simulink model "SAME5x_PIM_MCLV2_ioconfig"  (R2020b)
settings: Solver=FixedStepDiscrete  StartTime=0.0  StopTime=10.0  FixedStep=5e-5  RelTol=1e-3  EnableMultiTasking=on
InitFcn:
  | % DC Voltage
  | VDC = 24;
  | 
  | 
  | % QEI
  | lines = 4*1000;
  | p=4;
  | eleclines = lines/p;
  | inveleclines = 1/eleclines
undefined symbols (not defined in the file): AIN0, AIN6, DiscIntNeverNeededParam, gcbh, MCHP_CompilerOptimisation_Callback, MCHP_Master_Callback, MCHP_PDEC_Callback, MCHP_TCC_PWM_Callback, MCHP_UART_Config_Callback, PA02, PA03, PA06, PB08, Pin, VREFA
libraries: simulink x11, MCHP_Blockset x5
(part 3 of 3)

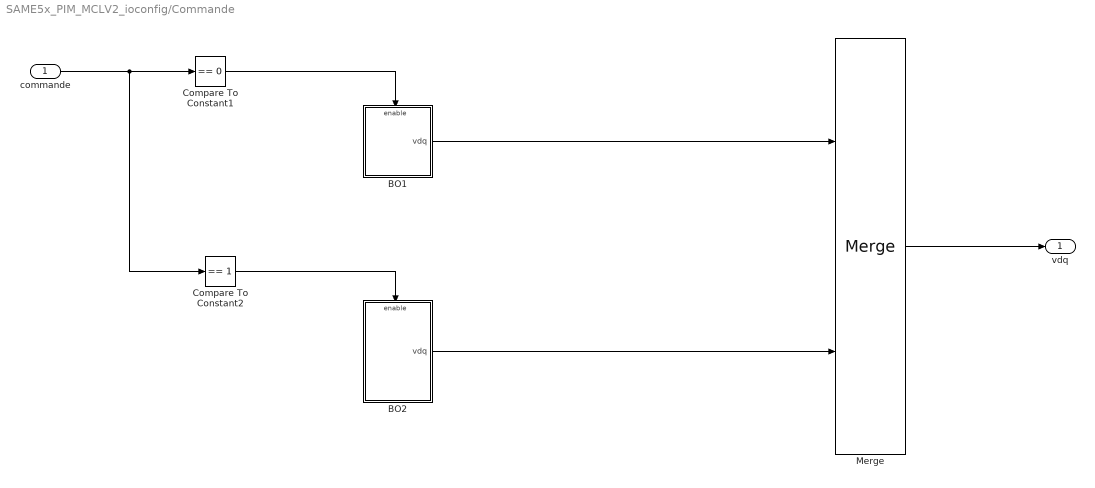
== system SAME5x_PIM_MCLV2_ioconfig/Commande ==
  commande : Inport
  BO1 : Subsystem
  BO2 : Subsystem
  Compare To Constant1 : simulink/Logic and Bit Operations/Compare To Constant  relop===  const=0  OutDataTypeStr=boolean
  Compare To Constant2 : simulink/Logic and Bit Operations/Compare To Constant  relop===  const=1  OutDataTypeStr=boolean
  Merge : Merge
  vdq : Outport  VectorParamsAs1DForOutWhenUnconnected=off
  wires:
  BO2/1(vdq) -> Merge/2
  BO1/1(vdq) -> Merge/1
  Compare To Constant2/1 -> BO2/Enable
  Merge/1 -> vdq/1
  commande/1 -> Compare To Constant2/1, Compare To Constant1/1
  Compare To Constant1/1 -> BO1/Enable

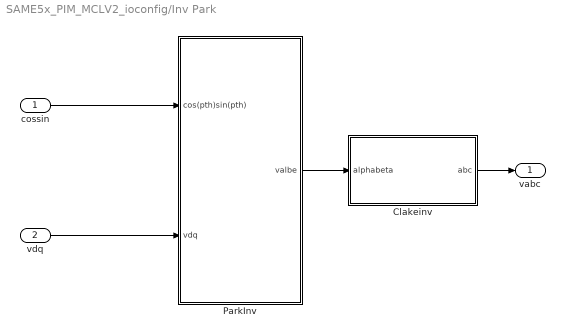
== system SAME5x_PIM_MCLV2_ioconfig/Inv Park ==
  cossin : Inport
  vdq : Inport  Port=2
  Clakeinv : Subsystem
  ParkInv : Subsystem
  vabc : Outport  VectorParamsAs1DForOutWhenUnconnected=off
  wires:
  Clakeinv/1(abc) -> vabc/1
  ParkInv/1(valbe) -> Clakeinv/1(alphabeta)
  cossin/1 -> ParkInv/1(cos(pth)sin(pth))
  vdq/1 -> ParkInv/2(vdq)

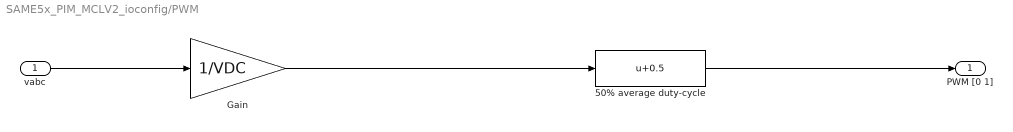
== system SAME5x_PIM_MCLV2_ioconfig/PWM ==
  vabc : Inport
  50% average duty-cycle : Bias  Bias=0.5
  Gain : Gain  Gain=1/VDC  OutDataTypeStr=double
  PWM [0 1] : Outport  VectorParamsAs1DForOutWhenUnconnected=off
  wires:
  Gain/1 -> 50% average duty-cycle/1
  50% average duty-cycle/1 -> PWM [0 1]/1
  vabc/1 -> Gain/1

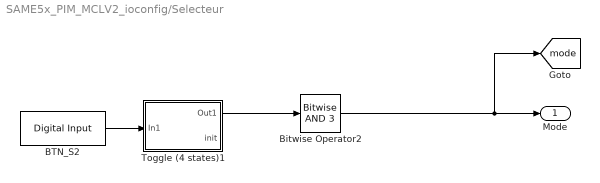
== system SAME5x_PIM_MCLV2_ioconfig/Selecteur ==
  BTN_S2 : MCHP_Blockset/Digital IO/Digital Input  PORT=Dynamic Options  PORT_TXT="D   [ 0  1  8  9  10  11  12  20  21 ]"  PIN=9  PACK=off  SIMULTANEOUS=off  ORDERING=None  SampleTime=.1  MCHP_PORT={Digital In}{DIN}2:0:D9;  MCHP_MASTERLINK=SAME5x_PIM_MCLV2_ioconfig/Microchip Master
      settings: SourceProductName=MPLAB Device Blocks for Simulink
  Bitwise Operator2 : simulink/Logic and Bit Operations/Bitwise Operator  logicop=AND  UseBitMask=on  BitMask=3  BitMaskRealWorld=Stored Integer
  Toggle (4 states)1 : Subsystem
  Mode : Outport  VectorParamsAs1DForOutWhenUnconnected=off
  tag scope: mode=global
  wires:
  BTN_S2/1 -> Toggle (4 states)1/1(In1)
  Toggle (4 states)1/1(Out1) -> Bitwise Operator2/1
  Bitwise Operator2/1 -> [mode], Mode/1

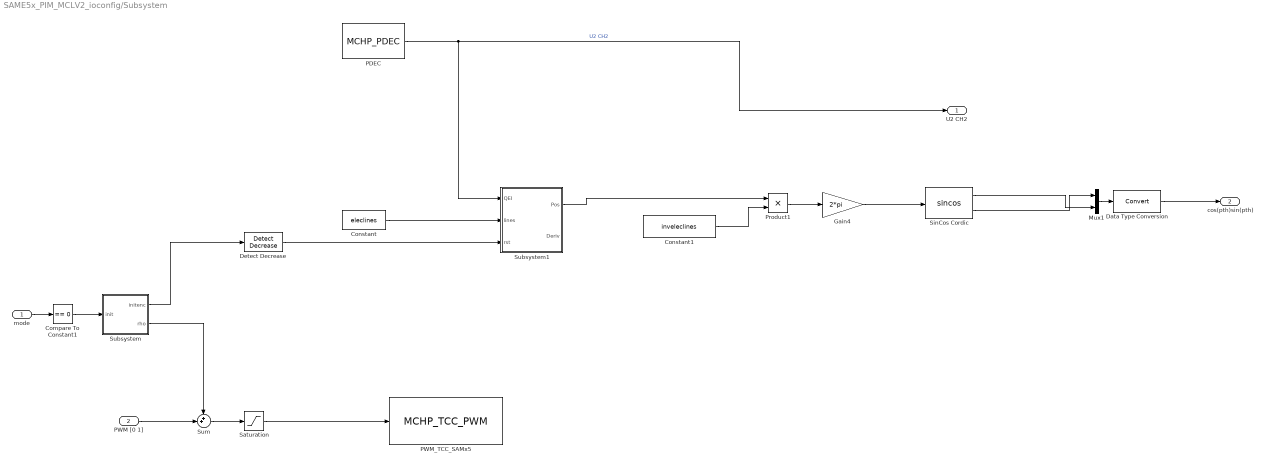
== system SAME5x_PIM_MCLV2_ioconfig/Subsystem ==
  mode : Inport
  PWM [0 1] : Inport  Port=2
  Compare To Constant1 : simulink/Logic and Bit Operations/Compare To Constant  relop===  const=0  OutDataTypeStr=boolean
  Constant : Constant  Value=eleclines
  Constant1 : Constant  Value=inveleclines
  Data Type Conversion : DataTypeConversion
  Detect Decrease : simulink/Logic and Bit Operations/Detect Decrease  vinit=0.0  OutDataTypeStr=boolean
  Gain4 : Gain  Gain=2*pi  OutMin=[0]  OutMax=[2*pi]  OutDataTypeStr=fixdt(0,16)
  Mux1 : Mux  Inputs=2
  PDEC : S-Function  InitFcn=MCHP_PDEC_Callback(gcb,'InitFcn');  FunctionName=MCHP_PDEC  Parameters=MCHP_PDEC_Callback(gcbh,'S_INPUT'),MCHP_PDEC_Callback(gcbh,'S_OUTPUT'),MCHP_PDEC_Callback(gcbh,'S_INPUT_Size'),MCHP_PDEC_Callback(gcbh,'S_OUTPUT_Size'),MCHP_PDEC_Callback(gcbh,'S_ListCustomDatatype'),SampleTime,0  SFunctionDeploymentMode=off  EnableBusSupport=off  mask(PDEC){Mode=Quadrature Encoder, index=Reset counter, QDI0=PC16 / Pin[70] / qdi0, QDI0_txt=Dynamic Options, QDI1=PC17 / Pin[71] / qdi1, QDI1_txt=Dynamic Options, QDI2=PC18 / Pin[72] / qdi2, QDI2_txt=Dynamic Options, maxCounterReset=-1, info=0, MCHP_MASTERLINK=SAME5x_PIM_MCLV2_ioconfig/Microchip Master, SampleTime=1e-4, MCHP_PORT={PDEC A}{PDEC_QDI0}5:0:P80;{PDEC B}{PDEC_QDI1}5:0:P81;{PDEC index}{PDEC_QDI2}5:0:P82;, MAXPOS_INPUT=off, RESET_INPUT=off, OutputCounter=on, OutputRevolution=off, CounterRevolution_length=Counter is 13 bits ; revolution is 3 bits, FILTER=2.55 (us)  ->  freq 196 (KHz), FILTER_TXT=2.55 (us)  ->  freq 196 (KHz), AutoCorrection=on, SWAP=off, QDI_invert_0=off, QDI_invert_1=off, QDI_invert_2=on}
      mask prompts: QDI0 "Phase A (QDI0)"; QDI0_txt "Signal 0"; QDI1 "Phase B (QDO1)"; QDI1_txt "Signal 1"; QDI2 "Index (QDI2)"; QDI2_txt "Signal 2"; maxCounterReset "Reset counter at value (-1 for never)"; SampleTime "Sample Time"; MAXPOS_INPUT "Max Counter is a block input"; RESET_INPUT "Reset Position and Counter on block input level"; OutputCounter "Output counter value"; OutputRevolution "Output revolution"; CounterRevolution_length "Length"; FILTER "Filter: min signal duration"; FILTER_TXT "Filter inputs"; AutoCorrection "Enable Auto-correction"; SWAP "Swap pin phase A && B"; QDI_invert_0 "Invert Phase A logic (QDI0)"; QDI_invert_1 "Invert Phase B logic (QDI1)"; QDI_invert_2 "Invert index logic (QDI2)"
      mask help:
      | PDEC peripheral for SAM D5x / E5x
      |
      | Quadrature Encoder
      mask init:
      | MCHP_PDEC_Callback(gcbh,'INITIALISATION');
      settings: CopyFcn=MCHP_Fun.BlockUpdate(gcbh);  DeleteFcn=MCHP_PDEC_Callback(gcbh,'DeleteFcn')  OpenFcn=MCHP_PDEC_Callback(gcb,'OPEN');
      mask TypeOptions Mode: Quadrature Encoder | Counter with direction
      mask Callback Mode: MCHP_PDEC_Callback(gcbh,'UpdateGUI');
      mask TypeOptions index: Not used | Reset counter
      mask Callback index: MCHP_PDEC_Callback(gcbh,'UpdateGUI');
      mask TypeOptions QDI0: PA24 / Pin[94] / qdi0 | PB18 / Pin[84] / qdi0 | PB23 / Pin[99] / qdi0 | PC16 / Pin[70] / qdi0
      mask TypeOptions QDI0_txt: Dynamic Options
      mask TypeOptions QDI1: PA25 / Pin[95] / qdi1 | PB19 / Pin[85] / qdi1 | PB24 / Pin[100] / qdi1 | PC17 / Pin[71] / qdi1
      mask TypeOptions QDI1_txt: Dynamic Options
      mask TypeOptions QDI2: PB20 / Pin[86] / qdi2 | PB22 / Pin[98] / qdi2 | PB25 / Pin[101] / qdi2 | PC18 / Pin[72] / qdi2
      mask TypeOptions QDI2_txt: Dynamic Options
      mask Callback MAXPOS_INPUT: MCHP_PDEC_Callback(gcbh,'UpdateGUI');
      mask Callback OutputRevolution: MCHP_PDEC_Callback(gcbh,'UpdateGUI');
      mask TypeOptions CounterRevolution_length: Counter is 16 bits ; no revolution | Counter is 15 bits ; revolution is 1 bit | Counter is 14 bits ; revolution is 2 bits | Counter is 13 bits ; revolution is 3 bits | Counter is 12 bits ; revolution is 4 bits | Counter is 11 bits ; revolution is 5 bits | Counter is 10 bits ; revolution is 6 bits | Counter is   9 bits ; revolution is 7 bits
      mask Callback CounterRevolution_length: MCHP_PDEC_Callback(gcbh,'UpdateGUI');
      mask TypeOptions FILTER: disabled | 10 (ns)  ->  freq 50 (MHz) | 20 (ns)  ->  freq 25 (MHz) | 30 (ns)  ->  freq 16.7 (MHz) | 40 (ns)  ->  freq 12.5 (MHz) | 50 (ns)  ->  freq 10 (MHz) | 60 (ns)  ->  freq 8.33 (MHz) | 70 (ns)  ->  freq 7.14 (MHz) | 80 (ns)  ->  freq 6.25 (MHz) | 90 (ns)  ->  freq 5.56 (MHz) | 100 (ns)  ->  freq 5 (MHz) | 110 (ns)  ->  freq 4.55 (MHz) | 120 (ns)  ->  freq 4.17 (MHz) | 130 (ns)  ->  freq 3.85 (MHz) | 140 (ns)  ->  freq 3.57 (MHz) | 150 (ns)  ->  freq 3.33 (MHz) | 160 (ns)  ->  freq 3.13 (MHz) | 170 (ns)  ->  freq 2.94 (MHz) | 180 (ns)  ->  freq 2.78 (MHz) | 190 (ns)  ->  freq 2.63 (MHz) | 200 (ns)  ->  freq 2.5 (MHz) | 210 (ns)  ->  freq 2.38 (MHz) | 220 (ns)  ->  freq 2.27 (MHz) | 230 (ns)  ->  freq 2.17 (MHz) | 240 (ns)  ->  freq 2.08 (MHz) | 250 (ns)  ->  freq 2 (MHz) | 260 (ns)  ->  freq 1.92 (MHz) | 270 (ns)  ->  freq 1.85 (MHz) | 280 (ns)  ->  freq 1.79 (MHz) | 290 (ns)  ->  freq 1.72 (MHz) | 300 (ns)  ->  freq 1.67 (MHz) | 310 (ns)  ->  freq 1.61 (MHz) | 320 (ns)  ->  freq 1.56 (MHz) | 330 (ns)  ->  freq 1.52 (MHz) | 340 (ns)  ->  freq 1.47 (MHz) | 350 (ns)  ->  freq 1.43 (MHz) | 360 (ns)  ->  freq 1.39 (MHz) | 370 (ns)  ->  freq 1.35 (MHz) | 380 (ns)  ->  freq 1.32 (MHz) | 390 (ns)  ->  freq 1.28 (MHz) | 400 (ns)  ->  freq 1.25 (MHz) | 410 (ns)  ->  freq 1.22 (MHz) | 420 (ns)  ->  freq 1.19 (MHz) | 430 (ns)  ->  freq 1.16 (MHz) | 440 (ns)  ->  freq 1.14 (MHz) | 450 (ns)  ->  freq 1.11 (MHz) | 460 (ns)  ->  freq 1.09 (MHz) | 470 (ns)  ->  freq 1.06 (MHz) | 480 (ns)  ->  freq 1.04 (MHz) | 490 (ns)  ->  freq 1.02 (MHz) | 500 (ns)  ->  freq 1e+03 (KHz) | 510 (ns)  ->  freq 980 (KHz) | 520 (ns)  ->  freq 962 (KHz) | 530 (ns)  ->  freq 943 (KHz) | 540 (ns)  ->  freq 926 (KHz) | 550 (ns)  ->  freq 909 (KHz) | 560 (ns)  ->  freq 893 (KHz) | 570 (ns)  ->  freq 877 (KHz) | 580 (ns)  ->  freq 862 (KHz) | 590 (ns)  ->  freq 847 (KHz) | 600 (ns)  ->  freq 833 (KHz) | 610 (ns)  ->  freq 820 (KHz) | 620 (ns)  ->  freq 806 (KHz) | 630 (ns)  ->  freq 794 (KHz) | 640 (ns)  ->  freq 781 (KHz) | 650 (ns)  ->  freq 769 (KHz) | 660 (ns)  ->  freq 758 (KHz) | 670 (ns)  ->  freq 746 (KHz) | 680 (ns)  ->  freq 735 (KHz) | 690 (ns)  ->  freq 725 (KHz) | 700 (ns)  ->  freq 714 (KHz) | 710 (ns)  ->  freq 704 (KHz) | 720 (ns)  ->  freq 694 (KHz) | 730 (ns)  ->  freq 685 (KHz) | 740 (ns)  ->  freq 676 (KHz) | 750 (ns)  ->  freq 667 (KHz) | 760 (ns)  ->  freq 658 (KHz) | 770 (ns)  ->  freq 649 (KHz) | 780 (ns)  ->  freq 641 (KHz) | 790 (ns)  ->  freq 633 (KHz) | 800 (ns)  ->  freq 625 (KHz) | 810 (ns)  ->  freq 617 (KHz) | 820 (ns)  ->  freq 610 (KHz) | 830 (ns)  ->  freq 602 (KHz) | 840 (ns)  ->  freq 595 (KHz) | 850 (ns)  ->  freq 588 (KHz) | 860 (ns)  ->  freq 581 (KHz) | 870 (ns)  ->  freq 575 (KHz) | 880 (ns)  ->  freq 568 (KHz) | 890 (ns)  ->  freq 562 (KHz) | 900 (ns)  ->  freq 556 (KHz) | 910 (ns)  ->  freq 549 (KHz) | 920 (ns)  ->  freq 543 (KHz) | 930 (ns)  ->  freq 538 (KHz) | 940 (ns)  ->  freq 532 (KHz) | 950 (ns)  ->  freq 526 (KHz) | 960 (ns)  ->  freq 521 (KHz) | 970 (ns)  ->  freq 515 (KHz) | 980 (ns)  ->  freq 510 (KHz) | 990 (ns)  ->  freq 505 (KHz) | 1e+03 (ns)  ->  freq 500 (KHz) | 1.01 (us)  ->  freq 495 (KHz) | 1.02 (us)  ->  freq 490 (KHz) | 1.03 (us)  ->  freq 485 (KHz) | 1.04 (us)  ->  freq 481 (KHz) | 1.05 (us)  ->  freq 476 (KHz) | 1.06 (us)  ->  freq 472 (KHz) | 1.07 (us)  ->  freq 467 (KHz) | 1.08 (us)  ->  freq 463 (KHz) | 1.09 (us)  ->  freq 459 (KHz) | 1.1 (us)  ->  freq 455 (KHz) | 1.11 (us)  ->  freq 450 (KHz) | 1.12 (us)  ->  freq 446 (KHz) | 1.13 (us)  ->  freq 442 (KHz) | 1.14 (us)  ->  freq 439 (KHz) | 1.15 (us)  ->  freq 435 (KHz) | 1.16 (us)  ->  freq 431 (KHz) | 1.17 (us)  ->  freq 427 (KHz) | 1.18 (us)  ->  freq 424 (KHz) | 1.19 (us)  ->  freq 420 (KHz) | 1.2 (us)  ->  freq 417 (KHz) | 1.21 (us)  ->  freq 413 (KHz) | 1.22 (us)  ->  freq 410 (KHz) | 1.23 (us)  ->  freq 407 (KHz) | 1.24 (us)  ->  freq 403 (KHz) | 1.25 (us)  ->  freq 400 (KHz) | 1.26 (us)  ->  freq 397 (KHz) | 1.27 (us)  ->  freq 394 (KHz) | 1.28 (us)  ->  freq 391 (KHz) | 1.29 (us)  ->  freq 388 (KHz) | 1.3 (us)  ->  freq 385 (KHz) | 1.31 (us)  ->  freq 382 (KHz) | 1.32 (us)  ->  freq 379 (KHz) | 1.33 (us)  ->  freq 376 (KHz) | 1.34 (us)  ->  freq 373 (KHz) | 1.35 (us)  ->  freq 370 (KHz) | 1.36 (us)  ->  freq 368 (KHz) | 1.37 (us)  ->  freq 365 (KHz) | 1.38 (us)  ->  freq 362 (KHz) | 1.39 (us)  ->  freq 360 (KHz) | 1.4 (us)  ->  freq 357 (KHz) | 1.41 (us)  ->  freq 355 (KHz) | 1.42 (us)  ->  freq 352 (KHz) | 1.43 (us)  ->  freq 350 (KHz) | 1.44 (us)  ->  freq 347 (KHz) | 1.45 (us)  ->  freq 345 (KHz) | 1.46 (us)  ->  freq 342 (KHz) | 1.47 (us)  ->  freq 340 (KHz) | 1.48 (us)  ->  freq 338 (KHz) | 1.49 (us)  ->  freq 336 (KHz) | 1.5 (us)  ->  freq 333 (KHz) | 1.51 (us)  ->  freq 331 (KHz) | 1.52 (us)  ->  freq 329 (KHz) | 1.53 (us)  ->  freq 327 (KHz) | 1.54 (us)  ->  freq 325 (KHz) | 1.55 (us)  ->  freq 323 (KHz) | 1.56 (us)  ->  freq 321 (KHz) | 1.57 (us)  ->  freq 318 (KHz) | 1.58 (us)  ->  freq 316 (KHz) | 1.59 (us)  ->  freq 314 (KHz) | 1.6 (us)  ->  freq 313 (KHz) | 1.61 (us)  ->  freq 311 (KHz) | 1.62 (us)  ->  freq 309 (KHz) | 1.63 (us)  ->  freq 307 (KHz) | 1.64 (us)  ->  freq 305 (KHz) | 1.65 (us)  ->  freq 303 (KHz) | 1.66 (us)  ->  freq 301 (KHz) | 1.67 (us)  ->  freq 299 (KHz) | 1.68 (us)  ->  freq 298 (KHz) | 1.69 (us)  ->  freq 296 (KHz) | 1.7 (us)  ->  freq 294 (KHz) | 1.71 (us)  ->  freq 292 (KHz) | 1.72 (us)  ->  freq 291 (KHz) | 1.73 (us)  ->  freq 289 (KHz) | 1.74 (us)  ->  freq 287 (KHz) | 1.75 (us)  ->  freq 286 (KHz) | 1.76 (us)  ->  freq 284 (KHz) | 1.77 (us)  ->  freq 282 (KHz) | 1.78 (us)  ->  freq 281 (KHz) | 1.79 (us)  ->  freq 279 (KHz) | 1.8 (us)  ->  freq 278 (KHz) | 1.81 (us)  ->  freq 276 (KHz) | 1.82 (us)  ->  freq 275 (KHz) | 1.83 (us)  ->  freq 273 (KHz) | 1.84 (us)  ->  freq 272 (KHz) | 1.85 (us)  ->  freq 270 (KHz) | 1.86 (us)  ->  freq 269 (KHz) | 1.87 (us)  ->  freq 267 (KHz) | 1.88 (us)  ->  freq 266 (KHz) | 1.89 (us)  ->  freq 265 (KHz) | 1.9 (us)  ->  freq 263 (KHz) | 1.91 (us)  ->  freq 262 (KHz) | 1.92 (us)  ->  freq 260 (KHz) | 1.93 (us)  ->  freq 259 (KHz) | 1.94 (us)  ->  freq 258 (KHz) | 1.95 (us)  ->  freq 256 (KHz) | 1.96 (us)  ->  freq 255 (KHz) | 1.97 (us)  ->  freq 254 (KHz) | 1.98 (us)  ->  freq 253 (KHz) | 1.99 (us)  ->  freq 251 (KHz) | 2 (us)  ->  freq 250 (KHz) | 2.01 (us)  ->  freq 249 (KHz) | 2.02 (us)  ->  freq 248 (KHz) | 2.03 (us)  ->  freq 246 (KHz) | 2.04 (us)  ->  freq 245 (KHz) | 2.05 (us)  ->  freq 244 (KHz) | 2.06 (us)  ->  freq 243 (KHz) | 2.07 (us)  ->  freq 242 (KHz) | 2.08 (us)  ->  freq 240 (KHz) | 2.09 (us)  ->  freq 239 (KHz) | 2.1 (us)  ->  freq 238 (KHz) | 2.11 (us)  ->  freq 237 (KHz) | 2.12 (us)  ->  freq 236 (KHz) | 2.13 (us)  ->  freq 235 (KHz) | 2.14 (us)  ->  freq 234 (KHz) | 2.15 (us)  ->  freq 233 (KHz) | 2.16 (us)  ->  freq 231 (KHz) | 2.17 (us)  ->  freq 230 (KHz) | 2.18 (us)  ->  freq 229 (KHz) | 2.19 (us)  ->  freq 228 (KHz) | 2.2 (us)  ->  freq 227 (KHz) | 2.21 (us)  ->  freq 226 (KHz) | 2.22 (us)  ->  freq 225 (KHz) | 2.23 (us)  ->  freq 224 (KHz) | 2.24 (us)  ->  freq 223 (KHz) | 2.25 (us)  ->  freq 222 (KHz) | 2.26 (us)  ->  freq 221 (KHz) | 2.27 (us)  ->  freq 220 (KHz) | 2.28 (us)  ->  freq 219 (KHz) | 2.29 (us)  ->  freq 218 (KHz) | 2.3 (us)  ->  freq 217 (KHz) | 2.31 (us)  ->  freq 216 (KHz) | 2.32 (us)  ->  freq 216 (KHz) | 2.33 (us)  ->  freq 215 (KHz) | 2.34 (us)  ->  freq 214 (KHz) | 2.35 (us)  ->  freq 213 (KHz) | 2.36 (us)  ->  freq 212 (KHz) | 2.37 (us)  ->  freq 211 (KHz) | 2.38 (us)  ->  freq 210 (KHz) | 2.39 (us)  ->  freq 209 (KHz) | 2.4 (us)  ->  freq 208 (KHz) | 2.41 (us)  ->  freq 207 (KHz) | 2.42 (us)  ->  freq 207 (KHz) | 2.43 (us)  ->  freq 206 (KHz) | 2.44 (us)  ->  freq 205 (KHz) | 2.45 (us)  ->  freq 204 (KHz) | 2.46 (us)  ->  freq 203 (KHz) | 2.47 (us)  ->  freq 202 (KHz) | 2.48 (us)  ->  freq 202 (KHz) | 2.49 (us)  ->  freq 201 (KHz) | 2.5 (us)  ->  freq 200 (KHz) | 2.51 (us)  ->  freq 199 (KHz) | 2.52 (us)  ->  freq 198 (KHz) | 2.53 (us)  ->  freq 198 (KHz) | 2.54 (us)  ->  freq 197 (KHz) | 2.55 (us)  ->  freq 196 (KHz)
      mask DialogControl ParameterGroupVar0 Prompt: Main
      mask DialogControl ParameterGroupVar2_copy Prompt: Inputs
      mask DialogControl ParameterGroupVar2 Prompt: Outputs
      mask DialogControl ParameterGroupVar1 Prompt: Options
      mask Display:
      | MCHP_DrawLogo;fprintf('PDEC\nQEI');
      | port_label('output',1,'POS');
  PWM_TCC_SAMx5 : S-Function  InitFcn=MCHP_TCC_PWM_Callback(gcb,'InitFcn');  FunctionName=MCHP_TCC_PWM  Parameters=MCHP_TCC_PWM_Callback(gcbh,'S_INPUT'),MCHP_TCC_PWM_Callback(gcbh,'S_OUTPUT'),MCHP_TCC_PWM_Callback(gcbh,'S_INPUT_Size'),MCHP_TCC_PWM_Callback(gcbh,'S_OUTPUT_Size'),MCHP_TCC_PWM_Callback(gcbh,'S_ListCustomDatatype'),SampleTime,0  SFunctionDeploymentMode=off  EnableBusSupport=off  mask(PWM - TCC){TCCREF=TCC 0, WAVE_choice=Center aligned PWM, MaxPeriod_s=5e-5, OTMX=Default, WO0=PA08 / Pin[33] / wo0, WO0_TXT=PA08 / Pin[33] / wo0, WO1=PA09 / Pin[34] / wo1, WO1_TXT=PA09 / Pin[34] / wo1, WO2=PA10 / Pin[35] / wo2, WO2_TXT=PA10 / Pin[35] / wo2, WO3=Not Used, WO3_TXT=Not Used, WO4=PA16 / Pin[66] / wo4, WO4_TXT=PA16 / Pin[66] / wo4, WO5=PA17 / Pin[67] / wo5, WO5_TXT=PA17 / Pin[67] / wo5, WO6=PA18 / Pin[68] / wo6, WO6_TXT=PA18 / Pin[68] / wo6, WO7=Not Used, WO7_TXT=Not Used, info=0, evalin_ws=PWM0max=MCHP_Fun.Hex2num('40A3860000000000');PWM0max=MCHP_Fun.Hex2num('40A3860000000000');PWM0max=MCHP_Fun.Hex2num('40A3860000000000');, SampleTime=1e-4, MCHP_PORT={PWM0_H0}{TCC0_WO0}5:1:P8;{PWM0_H1}{TCC0_WO1}5:1:P9;{PWM0_H2}{TCC0_WO2}5:1:P10;{PWM0_L0}{TCC0_WO4}5:1:P16;{PWM0_L1}{TCC0_WO5}5:1:P17;{PWM0_L2}{TCC0_WO6}5:1:P18;, MCHP_MASTERLINK=SAME5x_PIM_MCLV2_ioconfig/Microchip Master, INVEN_WO0=off, INVEN_WO1=off, INVEN_WO2=off, INVEN_WO3=off, INVEN_WO4=off, INVEN_WO5=off, INVEN_WO6=off, INVEN_WO7=off, SWAP_PWM0=off, SWAP_PWM1=off, SWAP_PWM2=off, SWAP_PWM3=off, POL_PWM0=off, POL_PWM1=off, POL_PWM2=off, POL_PWM3=off, POL_PWM4=off, POL_PWM5=off, InitPeriod_s=5e-5, InitDutyCycle_s=0.5, InitDeadTimeH_s=0.5e-6, InitDeadTimeL_s=0.5e-6, BlockInput_VectorScalar=Vectors (grouped by function), BlockInput_Period=Not a block input, BlockInput_DutyCycle=a Floating Point input within range [0 1], BlockInput_DeadTime=Not a block input}
      mask prompts: TCCREF "Select Pulse Width Modulation (PWM) Controller"; WAVE_choice "Generate signal"; MaxPeriod_s "Max period (s)  PWM0max = 2^11.29 (2499) for 5e-05s"; OTMX "Output Mapping matrix"; WO0 "Pin WO0 - PWM0_H0"; WO0_TXT "output pin WO0"; WO1 "Pin WO1 - PWM0_H1"; WO1_TXT "output pin WO1"; WO2 "Pin WO2 - PWM0_H2"; WO2_TXT "output pin WO2"; WO3 "Pin WO3 - PWM0_H3"; WO3_TXT "output pin WO3"; WO4 "Pin WO4 - PWM0_L0"; WO4_TXT "output pin WO4"; WO5 "Pin WO5 - PWM0_L1"; WO5_TXT "output pin WO5"; WO6 "Pin WO6 - PWM0_L2"; WO6_TXT "output pin WO6"; WO7 "Pin WO7 - PWM0_L3"; WO7_TXT "output pin WO7"; SampleTime "Sample Time"; INVEN_WO0 "Invert WO0 - PWM0_H0 output"; INVEN_WO1 "Invert WO1 - PWM0_H1 output"; INVEN_WO2 "Invert WO2 - PWM0_H2 output"; INVEN_WO3 "Invert WO3 output"; INVEN_WO4 "Invert WO4 - PWM0_L0 output"; INVEN_WO5 "Invert WO5 - PWM0_L1 output"; INVEN_WO6 "Invert WO6 - PWM0_L2 output"; INVEN_WO7 "Invert WO7 output"; SWAP_PWM0 "SWAP PWM0 High-Low side"; SWAP_PWM1 "SWAP PWM1 High-Low side"; SWAP_PWM2 "SWAP PWM2 High-Low side"; SWAP_PWM3 "SWAP PWM3 High-Low side"; POL_PWM0 "Reverse PWM0 polarity"; POL_PWM1 "Reverse PWM1 polarity"; POL_PWM2 "Reverse PWM2 polarity"; POL_PWM3 "Reverse PWM3 polarity"; POL_PWM4 "Reverse PWM4 polarity"; POL_PWM5 "Reverse PWM5 polarity"; InitPeriod_s "Initial Period (in s)"; InitDutyCycle_s "Initial Duty Cycle (in s)"; InitDeadTimeH_s "Initial Dead-time for PWMHx (in s)"; InitDeadTimeL_s "Initial Dead-time for PWMLx (in s)"; BlockInput_VectorScalar "Block input format"; BlockInput_Period "Period"; BlockInput_DutyCycle "Duty Cycle"; BlockInput_DeadTime "Dead Time"
      mask help: PWM peripheral for SAM D5x / E5x
      mask init:
      | MCHP_TCC_PWM_Callback(gcbh,'INITIALISATION');
      settings: CopyFcn=MCHP_Fun.BlockUpdate(gcbh);  DeleteFcn=MCHP_TCC_PWM_Callback(gcbh,'DeleteFcn')  OpenFcn=MCHP_TCC_PWM_Callback(gcb,'OPEN');
      mask TypeOptions TCCREF: TCC 0 | TCC 1 | TCC 2 | TCC 3 | TCC 4
      mask Callback TCCREF: MCHP_TCC_PWM_Callback(gcbh,'UpdateGUI');
      mask TypeOptions WAVE_choice: Left aligned PWM | Center aligned PWM
      mask TypeOptions OTMX: Default | Variant 1 | Variant 2 | Variant 3
      mask Callback OTMX: MCHP_TCC_PWM_Callback(gcbh,'UpdateGUI');
      mask TypeOptions WO0: Not Used |  --- | PA08 / Pin[33] / wo0 | PA20 / Pin[88] / wo0 | PB12 / Pin[41] / wo0 | PC04 / Pin[27] / wo0 | PC10 / Pin[52] / wo0 | PC16 / Pin[70] / wo0
      mask TypeOptions WO1: Not Used |  --- | PA09 / Pin[34] / wo1 | PA21 / Pin[89] / wo1 | PB13 / Pin[42] / wo1 | PC11 / Pin[55] / wo1 | PC17 / Pin[71] / wo1 | PD08 / Pin[47] / wo1
      mask TypeOptions WO2: Not Used |  --- | PA10 / Pin[35] / wo2 | PA22 / Pin[92] / wo2 | PB14 / Pin[43] / wo2 | PC12 / Pin[56] / wo2 | PC18 / Pin[72] / wo2 | PD09 / Pin[48] / wo2
      mask TypeOptions WO3: Not Used |  --- | PA11 / Pin[36] / wo3 | PA23 / Pin[93] / wo3 | PB15 / Pin[44] / wo3 | PC13 / Pin[57] / wo3 | PC19 / Pin[73] / wo3 | PD10 / Pin[49] / wo3
      mask TypeOptions WO4: Not Used |  --- | PA16 / Pin[66] / wo4 | PB10 / Pin[39] / wo4 | PB16 / Pin[82] / wo4 | PC14 / Pin[58] / wo4 | PC20 / Pin[74] / wo4 | PD11 / Pin[50] / wo4
      mask TypeOptions WO5: Not Used |  --- | PA17 / Pin[67] / wo5 | PB11 / Pin[40] / wo5 | PB17 / Pin[83] / wo5 | PC15 / Pin[59] / wo5 | PC21 / Pin[75] / wo5 | PD12 / Pin[51] / wo5
      mask TypeOptions WO6: Not Used |  --- | PA12 / Pin[60] / wo6 | PA18 / Pin[68] / wo6 | PB30 / Pin[121] / wo6 | PC22 / Pin[76] / wo6
      mask TypeOptions WO7: Not Used |  --- | PA13 / Pin[61] / wo7 | PA19 / Pin[69] / wo7 | PB31 / Pin[122] / wo7 | PC23 / Pin[77] / wo7
      mask TypeOptions BlockInput_VectorScalar: Independent Scalar | Vectors (grouped by function)
      mask TypeOptions BlockInput_Period: Not a block input | a Uint raw input (PWMxmax variable represent max period) | a Floating Point input within range [0 1] | a Floating Point input within range [-1 1] | a Floating Point input with physical scaling in (s)
      mask TypeOptions BlockInput_DutyCycle: Not a block input | a Uint raw input (PWMxmax variable represent max period) | a Floating Point input within range [0 1] | a Floating Point input within range [-1 1] | a Floating Point input with physical scaling in (s)
      mask TypeOptions BlockInput_DeadTime: Not a block input | a Uint raw input (PWMxmax variable represent max period) | a Floating Point input within range [0 1] | a Floating Point input within range [-1 1] | a Floating Point input with physical scaling in (s)
      mask DialogControl ParameterGroupVar0 Prompt: Main
      mask DialogControl ParameterGroupVar2_copy Prompt: Signals
      mask DialogControl ParameterGroupVar2 Prompt: Initial Values
      mask DialogControl ParameterGroupVar1 Prompt: Block Inputs
      mask Display:
      | fprintf(['PWM\nTCC' TCCREF(4:end)]);
      | port_label('input',1,'DutyCycle[0 1 2]');
  Product1 : Product  OutMin=[0]  OutMax=[1]  OutDataTypeStr=fixdt(1,16)
  Saturation : Saturate  UpperLimit=1  LowerLimit=0  LinearizeAsGain=off  OutDataTypeStr=double
  SinCos Cordic : Trigonometry  Operator=sincos  ApproximationMethod=CORDIC  NumberOfIterations=16
  Subsystem : Subsystem
  Subsystem1 : Subsystem
  Sum : Sum  Inputs=++|
  U2 CH2 : Outport
  cos(pth)sin(pth) : Outport  Port=2  VectorParamsAs1DForOutWhenUnconnected=off
  wires:
  PDEC/1 -> Subsystem1/1(QEI), U2 CH2/1  "U2 CH2"
  Mux1/1 -> Data Type Conversion/1
  Product1/1 -> Gain4/1
  SinCos Cordic/1 -> Mux1/2
  Constant1/1 -> Product1/2
  SinCos Cordic/2 -> Mux1/1
  Subsystem1/1(Pos) -> Product1/1
  Gain4/1 -> SinCos Cordic/1
  Sum/1 -> Saturation/1
  Subsystem/1(initenc) -> Detect Decrease/1
  PWM [0 1]/1 -> Sum/2
  mode/1 -> Compare To Constant1/1
  Constant/1 -> Subsystem1/2(lines)
  Detect Decrease/1 -> Subsystem1/3(rst)
  Compare To Constant1/1 -> Subsystem/1(init)
  Saturation/1 -> PWM_TCC_SAMx5/1
  Subsystem/2(rho) -> Sum/1
  Data Type Conversion/1 -> cos(pth)sin(pth)/1

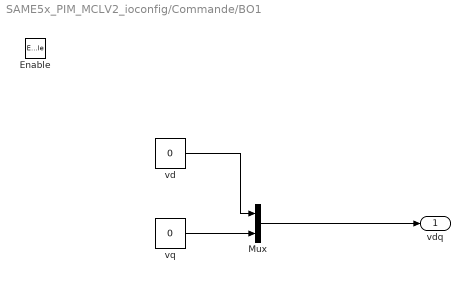
== system SAME5x_PIM_MCLV2_ioconfig/Commande/BO1 ==
  Enable : EnablePort
  Mux : Mux  Inputs=2
  vd : Constant  Value=0  OutMin=[-12]  OutMax=[12]  OutDataTypeStr=fixdt(1,16)
  vq : Constant  Value=0  OutMin=[-12]  OutMax=[12]  OutDataTypeStr=fixdt(1,16)
  vdq : Outport  VectorParamsAs1DForOutWhenUnconnected=off
  wires:
  vq/1 -> Mux/2
  Mux/1 -> vdq/1
  vd/1 -> Mux/1

== system SAME5x_PIM_MCLV2_ioconfig/Commande/BO2 ==
  Enable : EnablePort
  vd : Constant  Value=[0;2]  OutMin=[-12]  OutMax=[12]  OutDataTypeStr=fixdt(1,16)
  vdq : Outport  VectorParamsAs1DForOutWhenUnconnected=off
  wires:
  vd/1 -> vdq/1

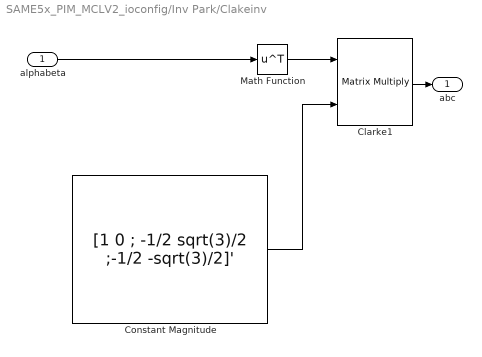
== system SAME5x_PIM_MCLV2_ioconfig/Inv Park/Clakeinv ==
  alphabeta : Inport
  Clarke1 : Product  Multiplication=Matrix(*)  RndMeth=Simplest  OutDataTypeStr=Inherit: Same as first input
  Constant Magnitude : Constant  Value=[1 0 ; -1/2 sqrt(3)/2 ;-1/2 -sqrt(3)/2]'  OutDataTypeStr=Inherit: Inherit via back propagation  SampleTime=-1
  Math Function : Math  Operator=transpose  SignedPower=on  SaturateOnIntegerOverflow=on
  abc : Outport  VectorParamsAs1DForOutWhenUnconnected=off
  wires:
  Clarke1/1 -> abc/1
  Math Function/1 -> Clarke1/1
  Constant Magnitude/1 -> Clarke1/2
  alphabeta/1 -> Math Function/1

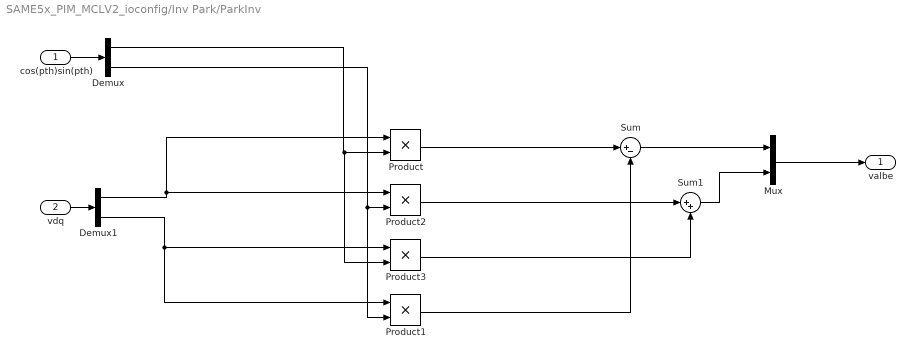
== system SAME5x_PIM_MCLV2_ioconfig/Inv Park/ParkInv ==
  cos(pth)sin(pth) : Inport
  vdq : Inport  Port=2
  Demux : Demux  Outputs=2
  Demux1 : Demux  Outputs=2
  Mux : Mux  Inputs=2
  Product{,1..3} (4 alike) : Product
  Sum : Sum  Inputs=|+-
  Sum1 : Sum  Inputs=|++
  valbe : Outport  VectorParamsAs1DForOutWhenUnconnected=off
  wires:
  Product3/1 -> Sum1/2
  Product2/1 -> Sum1/1
  Mux/1 -> valbe/1
  Demux/2 -> Product1/2, Product2/2
  Demux/1 -> Product/2, Product3/2
  Product/1 -> Sum/1
  Product1/1 -> Sum/2
  Sum1/1 -> Mux/2
  Demux1/2 -> Product1/1, Product3/1
  Demux1/1 -> Product/1, Product2/1
  Sum/1 -> Mux/1
  cos(pth)sin(pth)/1 -> Demux/1
  vdq/1 -> Demux1/1

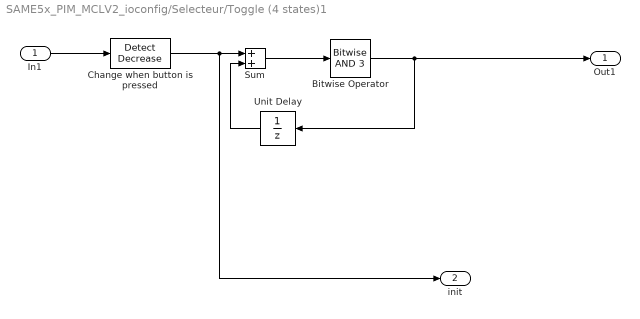
== system SAME5x_PIM_MCLV2_ioconfig/Selecteur/Toggle (4 states)1 ==
  In1 : Inport
  Bitwise Operator : simulink/Logic and Bit Operations/Bitwise Operator  logicop=AND  UseBitMask=on  BitMask=3  BitMaskRealWorld=Stored Integer
  Change when button is pressed : simulink/Logic and Bit Operations/Detect Decrease  vinit=0.0  OutDataTypeStr=uint8
  Sum : Sum  AccumDataTypeStr=uint16  OutDataTypeStr=uint16
  Unit Delay : UnitDelay  SampleTime=-1  HasFrameUpgradeWarning=on
  Out1 : Outport  VectorParamsAs1DForOutWhenUnconnected=off
  init : Outport  Port=2  VectorParamsAs1DForOutWhenUnconnected=off
  wires:
  In1/1 -> Change when button is pressed/1
  Sum/1 -> Bitwise Operator/1
  Unit Delay/1 -> Sum/2
  Bitwise Operator/1 -> Unit Delay/1, Out1/1
  Change when button is pressed/1 -> init/1, Sum/1

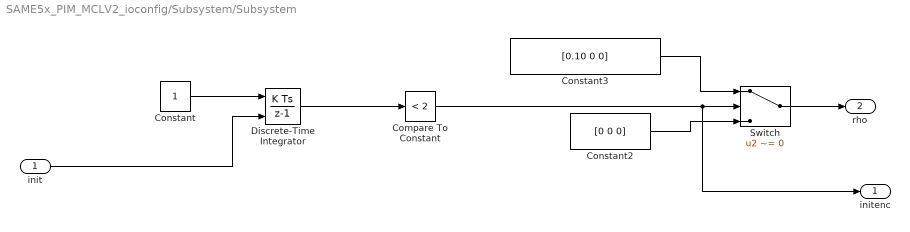
== system SAME5x_PIM_MCLV2_ioconfig/Subsystem/Subsystem ==
  init : Inport
  Compare To Constant : simulink/Logic and Bit Operations/Compare To Constant  relop=<  const=2  OutDataTypeStr=boolean
  Constant : Constant  OutDataTypeStr=double
  Constant2 : Constant  Value=[0 0 0]  OutDataTypeStr=double
  Constant3 : Constant  Value=[0.10 0 0]  OutDataTypeStr=double
  Discrete-Time Integrator : DiscreteIntegrator  ExternalReset=rising  SampleTime=1e-4  OutDataTypeStr=double  SaturateOnIntegerOverflow=on  UpperSaturationLimit=2  LowerSaturationLimit=0  ICPrevOutput=DiscIntNeverNeededParam  ICPrevScaledInput=DiscIntNeverNeededParam
  Switch : Switch  Criteria=u2 ~= 0
  initenc : Outport  VectorParamsAs1DForOutWhenUnconnected=off
  rho : Outport  Port=2  VectorParamsAs1DForOutWhenUnconnected=off
  wires:
  init/1 -> Discrete-Time Integrator/2
  Constant/1 -> Discrete-Time Integrator/1
  Discrete-Time Integrator/1 -> Compare To Constant/1
  Constant3/1 -> Switch/1
  Constant2/1 -> Switch/3
  Switch/1 -> rho/1
  Compare To Constant/1 -> initenc/1, Switch/2

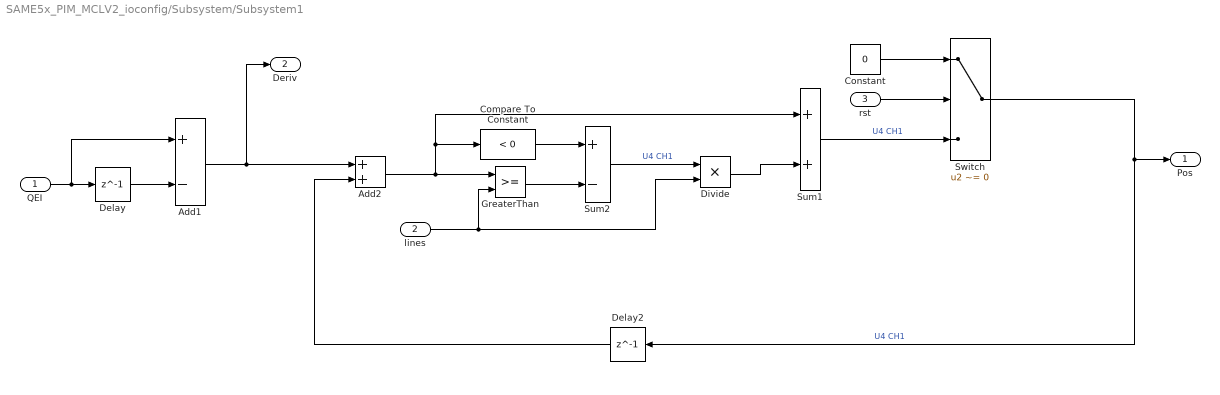
== system SAME5x_PIM_MCLV2_ioconfig/Subsystem/Subsystem1 ==
  QEI : Inport
  lines : Inport  Port=2
  rst : Inport  Port=3
  Add1 : Sum  Inputs=+-  OutDataTypeStr=Inherit: Same as accumulator
  Add2 : Sum  OutDataTypeStr=Inherit: Same as accumulator
  Compare To Constant : simulink/Logic and Bit Operations/Compare To Constant  relop=<  const=0  OutDataTypeStr=boolean
  Constant : Constant  Value=0  OutDataTypeStr=Inherit: Inherit via back propagation
  Delay : Delay  DelayLength=1  InitialCondition=0
  Delay2 : Delay  DelayLength=1  InitialCondition=0
  Divide : Product  Inputs=**  OutDataTypeStr=Inherit: Inherit via back propagation
  GreaterThan : RelationalOperator  OutDataTypeStr=boolean  RndMeth=Simplest
  Sum1 : Sum  InputSameDT=on  OutDataTypeStr=Inherit: Same as accumulator
  Sum2 : Sum  Inputs=+-  InputSameDT=on  AccumDataTypeStr=int16  OutDataTypeStr=Inherit: Same as accumulator
  Switch : Switch  Criteria=u2 ~= 0
  Pos : Outport
  Deriv : Outport  Port=2
  wires:
  Add1/1 -> Add2/1, Deriv/1
  Delay2/1 -> Add2/2
  Add2/1 -> GreaterThan/1, Sum1/1, Compare To Constant/1
  Switch/1 -> Delay2/1, Pos/1  "U4 CH1"
  Compare To Constant/1 -> Sum2/1
  QEI/1 -> Add1/1, Delay/1
  Delay/1 -> Add1/2
  Divide/1 -> Sum1/2
  rst/1 -> Switch/2
  Sum1/1 -> Switch/3  "U4 CH1"
  Constant/1 -> Switch/1
  GreaterThan/1 -> Sum2/2
  lines/1 -> GreaterThan/2, Divide/2
  Sum2/1 -> Divide/1  "U4 CH1"
